simulink model "zcu216_tut_spec_cx"  (R2025a)
(part 2 of 76)

      mask TypeOptions t228_ref_clk: 923.077 | 857.143 | 800 | 750 | 705.882 | 666.667 | 631.579 | 600 | 571.429 | 545.455 | 521.739 | 500 | 480 | 461.538 | 444.444 | 428.571 | 413.793 | 400 | 387.097 | 375 | 363.636 | 352.941 | 342.857 | 333.333 | 324.324 | 315.789 | 307.692 | 300 | 292.683 | 285.714 | 279.07 | 272.727 | 266.667 | 260.87 | 255.319 | 250 | 244.898 | 240 | 235.294 | 230.769 | 226.415 | 222.222 | 218.182 | 214.286 | 210.526 | 206.897 | 203.39 | 200 | 196.721 | 193.548 | 190.476 | 187.5 | 184.615 | 181.818 | 179.104 | 176.471 | 173.913 | 171.429 | 169.014 | 166.667 | 164.384 | 162.162 | 160 | 157.895 | 155.844 | 153.846 | 151.899 | 150 | 148.148 | 146.341 | 144.578 | 142.857 | 141.176 | 139.535 | 137.931 | 136.364 | 134.831 | 133.333 | 131.868 | 130.435 | 129.032 | 127.66 | 126.316 | 125 | 123.711 | 122.449 | 121.212 | 120 | 118.812 | 117.647 | 116.505 | 115.385 | 114.286 | 113.208 | 112.15 | 111.111 | 110.092 | 109.091 | 108.108 | 107.143 | 106.195 | 105.263 | 104.348 | 103.448 | 102.564
      mask Callback t228_QT_dac0_enable: enable_dac_opt(gcb,228,0,'QT');
      mask TypeOptions t228_QT_dac0_analog_output: Real | I/Q
      mask Callback t228_QT_dac0_analog_output:
      | validate_analog_data(gcb,228,0,'QT');
      | update_axis_clk(gcb,228);
      mask TypeOptions t228_QT_dac0_inter_mode: 1x | 2x | 3x | 4x | 5x | 6x | 8x | 10x | 12x | 16x | 20x | 24x | 40x
      mask Callback t228_QT_dac0_inter_mode:
      | % if I/Q output mode, need to copy interp factor before updating axis clk
      | % note only the even slice for the tile makes this check
      | if chk_param(gcb, 't228_QT_dac0_analog_output', 'I/Q')
      |   inter_mode = get_param(gcb, 't228_QT_dac0_inter_mode');
      |   set_param(gcb, 't228_QT_dac1_inter_mode', inter_mode);
      | end
      | 
      | update_axis_clk(gcb,228);
      mask TypeOptions t228_QT_dac0_sample_per_cycle: 4 | 5 | 6 | 7 | 8 | 9 | 10 | 11 | 12 | 13 | 14 | 15 | 16
      mask Callback t228_QT_dac0_sample_per_cycle:
      | % if I/Q output mode, need to copy samples per clk before updating axis clk
      | if chk_param(gcb, 't228_QT_dac0_analog_output', 'I/Q')
      |   spc = get_param(gcb, 't228_QT_dac0_sample_per_cycle');
      |   set_param(gcb, 't228_QT_dac1_sample_per_cycle', spc);
      | end
      | 
      | update_axis_clk_label(gcb,228);
      mask TypeOptions t228_QT_dac0_datapath_mode: DUC 0 to Fs/2
      mask TypeOptions t228_QT_dac0_mixer_type: Coarse | Fine
      mask Callback t228_QT_dac0_mixer_type: mixertype_callback(gcb,228,0,'QT');
      mask TypeOptions t228_QT_dac0_mixer_mode: Real -> Real | I/Q -> Real
      mask Callback t228_QT_dac0_mixer_mode: mixer_callback(gcb,228,0,'QT');
      mask TypeOptions t228_QT_dac0_coarse_freq: 0
      mask TypeOptions t228_QT_dac0_nyquist_zone: Zone 1 | Zone 2
      mask TypeOptions t228_QT_dac0_decode_mode: SNR Optimized | Linearity Optimized
      mask Callback t228_QT_dac1_enable: enable_dac_opt(gcb,228,1,'QT');
      mask TypeOptions t228_QT_dac1_analog_output: Real | I/Q
      mask Callback t228_QT_dac1_analog_output:
      | validate_analog_data(gcb,228,1,'QT');
      | update_axis_clk(gcb,228);
      mask TypeOptions t228_QT_dac1_inter_mode: 1x | 2x | 3x | 4x | 5x | 6x | 8x | 10x | 12x | 16x | 20x | 24x | 40x
      mask Callback t228_QT_dac1_inter_mode: update_axis_clk(gcb,228);
      mask TypeOptions t228_QT_dac1_sample_per_cycle: 4 | 5 | 6 | 7 | 8 | 9 | 10 | 11 | 12 | 13 | 14 | 15 | 16
      mask Callback t228_QT_dac1_sample_per_cycle: update_axis_clk_label(gcb,228);
      mask TypeOptions t228_QT_dac1_datapath_mode: DUC 0 to Fs/2
      mask TypeOptions t228_QT_dac1_mixer_type: Coarse | Fine
      mask Callback t228_QT_dac1_mixer_type: mixertype_callback(gcb,228,1,'QT');
      mask TypeOptions t228_QT_dac1_mixer_mode: Real -> Real | I/Q -> Real
      mask Callback t228_QT_dac1_mixer_mode: mixer_callback(gcb,228,1,'QT')
      mask TypeOptions t228_QT_dac1_coarse_freq: 0
      mask TypeOptions t228_QT_dac1_nyquist_zone: Zone 1 | Zone 2
      mask TypeOptions t228_QT_dac1_decode_mode: SNR Optimized | Linearity Optimized
      mask Callback t228_QT_dac2_enable: enable_dac_opt(gcb,228,2,'QT');
      mask TypeOptions t228_QT_dac2_analog_output: Real | I/Q
      mask Callback t228_QT_dac2_analog_output:
      | validate_analog_data(gcb,228,2,'QT');
      | update_axis_clk(gcb,228);
      mask TypeOptions t228_QT_dac2_inter_mode: 1x | 2x | 3x | 4x | 5x | 6x | 8x | 10x | 12x | 16x | 20x | 24x | 40x
      mask Callback t228_QT_dac2_inter_mode:
      | % if I/Q output mode, need to copy interp factor before updating axis clk
      | % note only the even slice for the tile makes this check
      | if chk_param(gcb, 't228_QT_dac2_analog_output', 'I/Q')
      |   inter_mode = get_param(gcb, 't228_QT_dac2_inter_mode');
      |   set_param(gcb, 't228_QT_dac3_inter_mode', inter_mode);
      | end
      | update_axis_clk(gcb,228);
      mask TypeOptions t228_QT_dac2_sample_per_cycle: 4 | 5 | 6 | 7 | 8 | 9 | 10 | 11 | 12 | 13 | 14 | 15 | 16
      mask Callback t228_QT_dac2_sample_per_cycle:
      | % if I/Q output mode, need to copy samples per clk before updating axis clk
      | % note only the even slice for the tile makes this check
      | if chk_param(gcb, 't228_QT_dac2_analog_output', 'I/Q')
      |   spc = get_param(gcb, 't228_QT_dac2_sample_per_cycle');
      |   set_param(gcb, 't228_QT_dac3_sample_per_cycle', spc);
      | end
      | update_axis_clk_label(gcb,228);
      mask TypeOptions t228_QT_dac2_datapath_mode: DUC 0 to Fs/2
      mask TypeOptions t228_QT_dac2_mixer_type: Coarse | Fine
      mask Callback t228_QT_dac2_mixer_type: mixertype_callback(gcb,228,2,'QT');
      mask TypeOptions t228_QT_dac2_mixer_mode: Real -> Real | I/Q -> Real
      mask Callback t228_QT_dac2_mixer_mode: mixer_callback(gcb,228,2,'QT')
      mask TypeOptions t228_QT_dac2_coarse_freq: 0
      mask TypeOptions t228_QT_dac2_nyquist_zone: Zone 1 | Zone 2
      mask TypeOptions t228_QT_dac2_decode_mode: SNR Optimized | Linearity Optimized
      mask Callback t228_QT_dac3_enable: enable_dac_opt(gcb,228,3,'QT');
      mask TypeOptions t228_QT_dac3_analog_output: Real | I/Q
      mask Callback t228_QT_dac3_analog_output:
      | validate_analog_data(gcb,228,3,'QT');
      | update_axis_clk(gcb,228);
      mask TypeOptions t228_QT_dac3_inter_mode: 1x | 2x | 3x | 4x | 5x | 6x | 8x | 10x | 12x | 16x | 20x | 24x | 40x
      mask Callback t228_QT_dac3_inter_mode: update_axis_clk(gcb,228);
      mask TypeOptions t228_QT_dac3_sample_per_cycle: 4 | 5 | 6 | 7 | 8 | 9 | 10 | 11 | 12 | 13 | 14 | 15 | 16
      mask Callback t228_QT_dac3_sample_per_cycle: update_axis_clk_label(gcb,228);
      mask TypeOptions t228_QT_dac3_datapath_mode: DUC 0 to Fs/2
      mask TypeOptions t228_QT_dac3_mixer_type: Coarse | Fine
      mask Callback t228_QT_dac3_mixer_type: mixertype_callback(gcb,228,3,'QT');
      mask TypeOptions t228_QT_dac3_mixer_mode: Real -> Real | I/Q -> Real
      mask Callback t228_QT_dac3_mixer_mode: mixer_callback(gcb,228,3,'QT')
      mask TypeOptions t228_QT_dac3_coarse_freq: 0
      mask TypeOptions t228_QT_dac3_nyquist_zone: Zone 1 | Zone 2
      mask TypeOptions t228_QT_dac3_decode_mode: SNR Optimized | Linearity Optimized
      mask Callback t228_DT_dac0_enable: enable_dac_opt(gcb,228,0,'DT');
      mask TypeOptions t228_DT_dac0_analog_output: Real | I/Q
      mask Callback t228_DT_dac0_analog_output:
      | validate_analog_data(gcb,228,0,'DT');
      | update_axis_clk(gcb,228);
      mask TypeOptions t228_DT_dac0_inter_mode: 1x | 2x | 3x | 4x | 5x | 6x | 8x | 10x | 12x | 16x | 20x | 24x | 40x
      mask Callback t228_DT_dac0_inter_mode:
      | % if I/Q output mode, need to copy interp factor before updating axis clk
      | % note only the even slice for the tile makes this check
      | if chk_param(gcb, 't228_DT_dac0_analog_output', 'I/Q')
      |   inter_mode = get_param(gcb, 't228_DT_dac0_inter_mode');
      |   set_param(gcb, 't228_DT_dac1_inter_mode', inter_mode);
      | end
      | 
      | update_axis_clk(gcb,228);
      mask TypeOptions t228_DT_dac0_sample_per_cycle: 4 | 5 | 6 | 7 | 8 | 9 | 10 | 11 | 12 | 13 | 14 | 15 | 16
      mask Callback t228_DT_dac0_sample_per_cycle:
      | % if I/Q output mode, need to copy samples per clk before updating axis clk
      | if chk_param(gcb, 't228_DT_dac0_analog_output', 'I/Q')
      |   spc = get_param(gcb, 't228_DT_dac0_sample_per_cycle');
      |   set_param(gcb, 't228_DT_dac1_sample_per_cycle', spc);
      | end
      | update_axis_clk_label(gcb,228);
      mask TypeOptions t228_DT_dac0_datapath_mode: DUC 0 to Fs/2
      mask TypeOptions t228_DT_dac0_mixer_type: Coarse | Fine
      mask Callback t228_DT_dac0_mixer_type: mixertype_callback(gcb,228,0,'DT');
      mask TypeOptions t228_DT_dac0_mixer_mode: Real -> Real | I/Q -> Real
      mask Callback t228_DT_dac0_mixer_mode: mixer_callback(gcb,228,0,'DT');
      mask TypeOptions t228_DT_dac0_coarse_freq: 0
      mask TypeOptions t228_DT_dac0_nyquist_zone: Zone 1 | Zone 2
      mask TypeOptions t228_DT_dac0_decode_mode: SNR Optimized | Linearity Optimized
      mask Callback t228_DT_dac1_enable: enable_dac_opt(gcb,228,1,'DT');
      mask TypeOptions t228_DT_dac1_analog_output: Real
      mask Callback t228_DT_dac1_analog_output:
      | validate_analog_data(gcb,228,1,'DT');
      | update_axis_clk(gcb,228);
      mask TypeOptions t228_DT_dac1_inter_mode: 1x | 2x | 3x | 4x | 5x | 6x | 8x | 10x | 12x | 16x | 20x | 24x | 40x
      mask Callback t228_DT_dac1_inter_mode: update_axis_clk(gcb,228);
      mask TypeOptions t228_DT_dac1_sample_per_cycle: 4 | 5 | 6 | 7 | 8 | 9 | 10 | 11 | 12 | 13 | 14 | 15 | 16
      mask Callback t228_DT_dac1_sample_per_cycle:
      | %update_axis_clk(gcb);
      | update_axis_clk_label(gcb,228);
      mask TypeOptions t228_DT_dac1_datapath_mode: DUC 0 to Fs/2
      mask TypeOptions t228_DT_dac1_mixer_type: Coarse | Fine
      mask Callback t228_DT_dac1_mixer_type: mixertype_callback(gcb,228,1,'DT');
      mask TypeOptions t228_DT_dac1_mixer_mode: Real -> Real | I/Q -> Real
      mask Callback t228_DT_dac1_mixer_mode: mixer_callback(gcb,228,1,'DT');
      mask TypeOptions t228_DT_dac1_coarse_freq: 0
      mask TypeOptions t228_DT_dac1_nyquist_zone: Zone 1 | Zone 2
      mask TypeOptions t228_DT_dac1_decode_mode: SNR Optimized | Linearity Optimized
      mask Callback t229_sample_rate: update_rfdc_clocking(gcb,229);
      mask TypeOptions t229_clk_out: 125 | 62.5 | 31.25 | 15.625
      mask Callback t229_enable_pll:
      | %update_rfdc_clocking(gcb);
      | update_pll(gcb,229);
      mask TypeOptions t229_ref_clk: 923.077 | 857.143 | 800 | 750 | 705.882 | 666.667 | 631.579 | 600 | 571.429 | 545.455 | 521.739 | 500 | 480 | 461.538 | 444.444 | 428.571 | 413.793 | 400 | 387.097 | 375 | 363.636 | 352.941 | 342.857 | 333.333 | 324.324 | 315.789 | 307.692 | 300 | 292.683 | 285.714 | 279.07 | 272.727 | 266.667 | 260.87 | 255.319 | 250 | 244.898 | 240 | 235.294 | 230.769 | 226.415 | 222.222 | 218.182 | 214.286 | 210.526 | 206.897 | 203.39 | 200 | 196.721 | 193.548 | 190.476 | 187.5 | 184.615 | 181.818 | 179.104 | 176.471 | 173.913 | 171.429 | 169.014 | 166.667 | 164.384 | 162.162 | 160 | 157.895 | 155.844 | 153.846 | 151.899 | 150 | 148.148 | 146.341 | 144.578 | 142.857 | 141.176 | 139.535 | 137.931 | 136.364 | 134.831 | 133.333 | 131.868 | 130.435 | 129.032 | 127.66 | 126.316 | 125 | 123.711 | 122.449 | 121.212 | 120 | 118.812 | 117.647 | 116.505 | 115.385 | 114.286 | 113.208 | 112.15 | 111.111 | 110.092 | 109.091 | 108.108 | 107.143 | 106.195 | 105.263 | 104.348 | 103.448 | 102.564
      mask Callback t229_QT_dac0_enable: enable_dac_opt(gcb,229,0,'QT');
      mask TypeOptions t229_QT_dac0_analog_output: Real | I/Q
      mask Callback t229_QT_dac0_analog_output:
      | validate_analog_data(gcb,229,0,'QT');
      | update_axis_clk(gcb,229);
      mask TypeOptions t229_QT_dac0_inter_mode: 1x | 2x | 3x | 4x | 5x | 6x | 8x | 10x | 12x | 16x | 20x | 24x | 40x
      mask Callback t229_QT_dac0_inter_mode:
      | % if I/Q output mode, need to copy interp factor before updating axis clk
      | % note only the even slice for the tile makes this check
      | if chk_param(gcb, 't229_QT_dac0_analog_output', 'I/Q')
      |   inter_mode = get_param(gcb, 't229_QT_dac0_inter_mode');
      |   set_param(gcb, 't229_QT_dac1_inter_mode', inter_mode);
      | end
      | update_axis_clk(gcb,229);
      mask TypeOptions t229_QT_dac0_sample_per_cycle: 4 | 5 | 6 | 7 | 8 | 9 | 10 | 11 | 12 | 13 | 14 | 15 | 16
      mask Callback t229_QT_dac0_sample_per_cycle:
      | % if I/Q output mode, need to copy samples per clk before updating axis clk
      | % note only the even slice for the tile makes this check
      | if chk_param(gcb, 't229_QT_dac0_analog_output', 'I/Q')
      |   spc = get_param(gcb, 't229_QT_dac0_sample_per_cycle');
      |   set_param(gcb, 't229_QT_dac1_sample_per_cycle', spc);
      | end
      | update_axis_clk_label(gcb,229);
      mask TypeOptions t229_QT_dac0_datapath_mode: DUC 0 to Fs/2
      mask TypeOptions t229_QT_dac0_mixer_type: Coarse | Fine
      mask Callback t229_QT_dac0_mixer_type: mixertype_callback(gcb,229,0,'QT');
      mask TypeOptions t229_QT_dac0_mixer_mode: Real -> Real | I/Q -> Real
      mask Callback t229_QT_dac0_mixer_mode: mixer_callback(gcb,229,0,'QT');
      mask TypeOptions t229_QT_dac0_coarse_freq: 0
      mask TypeOptions t229_QT_dac0_nyquist_zone: Zone 1 | Zone 2
      mask TypeOptions t229_QT_dac0_decode_mode: SNR Optimized | Linearity Optimized
      mask Callback t229_QT_dac1_enable: enable_dac_opt(gcb,229,1,'QT');
      mask TypeOptions t229_QT_dac1_analog_output: Real
      mask Callback t229_QT_dac1_analog_output:
      | validate_analog_data(gcb,229,1,'QT');
      | update_axis_clk(gcb,229);
      mask TypeOptions t229_QT_dac1_inter_mode: 1x | 2x | 3x | 4x | 5x | 6x | 8x | 10x | 12x | 16x | 20x | 24x | 40x
      mask Callback t229_QT_dac1_inter_mode: update_axis_clk(gcb,229);
      mask TypeOptions t229_QT_dac1_sample_per_cycle: 4 | 5 | 6 | 7 | 8 | 9 | 10 | 11 | 12 | 13 | 14 | 15 | 16
      mask Callback t229_QT_dac1_sample_per_cycle: update_axis_clk_label(gcb,229);
      mask TypeOptions t229_QT_dac1_datapath_mode: DUC 0 to Fs/2
      mask TypeOptions t229_QT_dac1_mixer_type: Coarse | Fine
      mask Callback t229_QT_dac1_mixer_type: mixertype_callback(gcb,229,1,'QT');
      mask TypeOptions t229_QT_dac1_mixer_mode: Real -> Real | I/Q -> Real
      mask Callback t229_QT_dac1_mixer_mode: mixer_callback(gcb,229,1,'QT')
      mask TypeOptions t229_QT_dac1_coarse_freq: 0
      mask TypeOptions t229_QT_dac1_nyquist_zone: Zone 1 | Zone 2
      mask TypeOptions t229_QT_dac1_decode_mode: SNR Optimized | Linearity Optimized
      mask Callback t229_QT_dac2_enable: enable_dac_opt(gcb,229,2,'QT');
      mask TypeOptions t229_QT_dac2_analog_output: Real | I/Q
      mask Callback t229_QT_dac2_analog_output:
      | validate_analog_data(gcb,229,2,'QT');
      | update_axis_clk(gcb,229);
      mask TypeOptions t229_QT_dac2_inter_mode: 1x | 2x | 3x | 4x | 5x | 6x | 8x | 10x | 12x | 16x | 20x | 24x | 40x
      mask Callback t229_QT_dac2_inter_mode:
      | % if I/Q output mode, need to copy interp factor before updating axis clk
      | % note only the even slice for the tile makes this check
      | if chk_param(gcb, 't229_QT_dac2_analog_output', 'I/Q')
      |   inter_mode = get_param(gcb, 't229_QT_dac2_inter_mode');
      |   set_param(gcb, 't229_QT_dac3_inter_mode', inter_mode);
      | end
      | update_axis_clk(gcb,229);
      mask TypeOptions t229_QT_dac2_sample_per_cycle: 4 | 5 | 6 | 7 | 8 | 9 | 10 | 11 | 12 | 13 | 14 | 15 | 16
      mask Callback t229_QT_dac2_sample_per_cycle:
      | % if I/Q output mode, need to copy samples per clk before updating axis clk
      | % note only the even slice for the tile makes this check
      | if chk_param(gcb, 't229_QT_dac2_analog_output', 'I/Q')
      |   spc = get_param(gcb, 't229_QT_dac2_sample_per_cycle');
      |   set_param(gcb, 't229_QT_dac3_sample_per_cycle', spc);
      | end
      | update_axis_clk_label(gcb,229);
      mask TypeOptions t229_QT_dac2_datapath_mode: DUC 0 to Fs/2
      mask TypeOptions t229_QT_dac2_mixer_type: Coarse | Fine
      mask Callback t229_QT_dac2_mixer_type: mixertype_callback(gcb,229,2,'QT');
      mask TypeOptions t229_QT_dac2_mixer_mode: Real -> Real | I/Q -> Real
      mask Callback t229_QT_dac2_mixer_mode: mixer_callback(gcb,229,2,'QT')
      mask TypeOptions t229_QT_dac2_coarse_freq: 0
      mask TypeOptions t229_QT_dac2_nyquist_zone: Zone 1 | Zone 2
      mask TypeOptions t229_QT_dac2_decode_mode: SNR Optimized | Linearity Optimized
      mask Callback t229_QT_dac3_enable: enable_dac_opt(gcb,229,3,'QT');
      mask TypeOptions t229_QT_dac3_analog_output: Real | I/Q
      mask Callback t229_QT_dac3_analog_output:
      | validate_analog_data(gcb,229,3,'QT');
      | update_axis_clk(gcb,229);
      mask TypeOptions t229_QT_dac3_inter_mode: 1x | 2x | 3x | 4x | 5x | 6x | 8x | 10x | 12x | 16x | 20x | 24x | 40x
      mask Callback t229_QT_dac3_inter_mode: update_axis_clk(gcb,229);
      mask TypeOptions t229_QT_dac3_sample_per_cycle: 4 | 5 | 6 | 7 | 8 | 9 | 10 | 11 | 12 | 13 | 14 | 15 | 16
      mask Callback t229_QT_dac3_sample_per_cycle: update_axis_clk_label(gcb,229);
      mask TypeOptions t229_QT_dac3_datapath_mode: DUC 0 to Fs/2
      mask TypeOptions t229_QT_dac3_mixer_type: Coarse | Fine
      mask Callback t229_QT_dac3_mixer_type: mixertype_callback(gcb,229,3,'QT');
      mask TypeOptions t229_QT_dac3_mixer_mode: Real -> Real | I/Q -> Real
      mask Callback t229_QT_dac3_mixer_mode: mixer_callback(gcb,229,3,'QT')
      mask TypeOptions t229_QT_dac3_coarse_freq: 0
      mask TypeOptions t229_QT_dac3_nyquist_zone: Zone 1 | Zone 2
      mask TypeOptions t229_QT_dac3_decode_mode: SNR Optimized | Linearity Optimized
      mask Callback t229_DT_dac0_enable: enable_dac_opt(gcb,229,0,'DT');
      mask TypeOptions t229_DT_dac0_analog_output: Real | I/Q
      mask Callback t229_DT_dac0_analog_output:
      | validate_analog_data(gcb,229,0,'DT');
      | update_axis_clk(gcb,229);
      mask TypeOptions t229_DT_dac0_inter_mode: 1x | 2x | 3x | 4x | 5x | 6x | 8x | 10x | 12x | 16x | 20x | 24x | 40x
      mask Callback t229_DT_dac0_inter_mode:
      | % if I/Q output mode, need to copy interp factor before updating axis clk
      | % note only the even slice for the tile makes this check
      | if chk_param(gcb, 't229_DT_dac0_analog_output', 'I/Q')
      |   inter_mode = get_param(gcb, 't229_DT_dac0_inter_mode');
      |   set_param(gcb, 't229_DT_dac1_inter_mode', inter_mode);
      | end
      | update_axis_clk(gcb,229);
      mask TypeOptions t229_DT_dac0_sample_per_cycle: 4 | 5 | 6 | 7 | 8 | 9 | 10 | 11 | 12 | 13 | 14 | 15 | 16
      mask Callback t229_DT_dac0_sample_per_cycle:
      | % if I/Q output mode, need to copy samples per clk before updating axis clk
      | % note only the even slice for the tile makes this check
      | if chk_param(gcb, 't229_DT_dac0_analog_output', 'I/Q')
      |   spc = get_param(gcb, 't229_DT_dac0_sample_per_cycle');
      |   set_param(gcb, 't229_DT_dac1_sample_per_cycle', spc);
      | end
      | update_axis_clk_label(gcb,229);
      mask TypeOptions t229_DT_dac0_datapath_mode: DUC 0 to Fs/2
      mask TypeOptions t229_DT_dac0_mixer_type: Coarse | Fine
      mask Callback t229_DT_dac0_mixer_type: mixertype_callback(gcb,229,0,'DT');
      mask TypeOptions t229_DT_dac0_mixer_mode: Real -> Real | I/Q -> Real
      mask Callback t229_DT_dac0_mixer_mode: mixer_callback(gcb,229,0,'DT');
      mask TypeOptions t229_DT_dac0_coarse_freq: 0
      mask TypeOptions t229_DT_dac0_nyquist_zone: Zone 1 | Zone 2
      mask TypeOptions t229_DT_dac0_decode_mode: SNR Optimized | Linearity Optimized
      mask Callback t229_DT_dac1_enable: enable_dac_opt(gcb,229,1,'DT');
      mask TypeOptions t229_DT_dac1_analog_output: Real
      mask Callback t229_DT_dac1_analog_output:
      | validate_analog_data(gcb,229,1,'DT');
      | update_axis_clk(gcb,229);
      mask TypeOptions t229_DT_dac1_inter_mode: 1x | 2x | 3x | 4x | 5x | 6x | 8x | 10x | 12x | 16x | 20x | 24x | 40x
      mask Callback t229_DT_dac1_inter_mode: update_axis_clk(gcb,229);
      mask TypeOptions t229_DT_dac1_sample_per_cycle: 4 | 5 | 6 | 7 | 8 | 9 | 10 | 11 | 12 | 13 | 14 | 15 | 16
      mask Callback t229_DT_dac1_sample_per_cycle:
      | %update_axis_clk(gcb);
      | update_axis_clk_label(gcb,229);
      mask TypeOptions t229_DT_dac1_datapath_mode: DUC 0 to Fs/2
      mask TypeOptions t229_DT_dac1_mixer_type: Coarse | Fine
      mask Callback t229_DT_dac1_mixer_type: mixertype_callback(gcb,229,1,'DT');
      mask TypeOptions t229_DT_dac1_mixer_mode: Real -> Real | I/Q -> Real
      mask Callback t229_DT_dac1_mixer_mode: mixer_callback(gcb,229,1,'DT');
      mask TypeOptions t229_DT_dac1_coarse_freq: 0
      mask TypeOptions t229_DT_dac1_nyquist_zone: Zone 1 | Zone 2
      mask TypeOptions t229_DT_dac1_decode_mode: SNR Optimized | Linearity Optimized
      mask Callback t230_sample_rate: update_rfdc_clocking(gcb,230);
      mask TypeOptions t230_clk_out: 125 | 62.5 | 31.25 | 15.625
      mask Callback t230_enable_pll:
      | %update_rfdc_clocking(gcb);
      | update_pll(gcb,230);
      mask TypeOptions t230_ref_clk: 923.077 | 857.143 | 800 | 750 | 705.882 | 666.667 | 631.579 | 600 | 571.429 | 545.455 | 521.739 | 500 | 480 | 461.538 | 444.444 | 428.571 | 413.793 | 400 | 387.097 | 375 | 363.636 | 352.941 | 342.857 | 333.333 | 324.324 | 315.789 | 307.692 | 300 | 292.683 | 285.714 | 279.07 | 272.727 | 266.667 | 260.87 | 255.319 | 250 | 244.898 | 240 | 235.294 | 230.769 | 226.415 | 222.222 | 218.182 | 214.286 | 210.526 | 206.897 | 203.39 | 200 | 196.721 | 193.548 | 190.476 | 187.5 | 184.615 | 181.818 | 179.104 | 176.471 | 173.913 | 171.429 | 169.014 | 166.667 | 164.384 | 162.162 | 160 | 157.895 | 155.844 | 153.846 | 151.899 | 150 | 148.148 | 146.341 | 144.578 | 142.857 | 141.176 | 139.535 | 137.931 | 136.364 | 134.831 | 133.333 | 131.868 | 130.435 | 129.032 | 127.66 | 126.316 | 125 | 123.711 | 122.449 | 121.212 | 120 | 118.812 | 117.647 | 116.505 | 115.385 | 114.286 | 113.208 | 112.15 | 111.111 | 110.092 | 109.091 | 108.108 | 107.143 | 106.195 | 105.263 | 104.348 | 103.448 | 102.564
      mask Callback t230_QT_dac0_enable: enable_dac_opt(gcb,230,0,'QT');
      mask TypeOptions t230_QT_dac0_analog_output: Real | I/Q
      mask Callback t230_QT_dac0_analog_output:
      | validate_analog_data(gcb,230,0,'QT');
      | update_axis_clk(gcb,230);
      mask TypeOptions t230_QT_dac0_inter_mode: 1x | 2x | 3x | 4x | 5x | 6x | 8x | 10x | 12x | 16x | 20x | 24x | 40x
      mask Callback t230_QT_dac0_inter_mode:
      | % if I/Q output mode, need to copy interp factor before updating axis clk
      | % note only the even slice for the tile makes this check
      | if chk_param(gcb, 't230_QT_dac0_analog_output', 'I/Q')
      |   inter_mode = get_param(gcb, 't230_QT_dac0_inter_mode');
      |   set_param(gcb, 't230_QT_dac1_inter_mode', inter_mode);
      | end
      | update_axis_clk(gcb,230);
      mask TypeOptions t230_QT_dac0_sample_per_cycle: 4 | 5 | 6 | 7 | 8 | 9 | 10 | 11 | 12 | 13 | 14 | 15 | 16
      mask Callback t230_QT_dac0_sample_per_cycle:
      | % if I/Q output mode, need to copy samples per clk before updating axis clk
      | % note only the even slice for the tile makes this check
      | if chk_param(gcb, 't230_QT_dac0_analog_output', 'I/Q')
      |   spc = get_param(gcb, 't230_QT_dac0_sample_per_cycle');
      |   set_param(gcb, 't230_QT_dac1_sample_per_cycle', spc);
      | end
      | 
      | update_axis_clk_label(gcb,230);
      mask TypeOptions t230_QT_dac0_datapath_mode: DUC 0 to Fs/2
      mask TypeOptions t230_QT_dac0_mixer_type: Coarse | Fine
      mask Callback t230_QT_dac0_mixer_type: mixertype_callback(gcb,230,0,'QT');
      mask TypeOptions t230_QT_dac0_mixer_mode: Real -> Real | I/Q -> Real
      mask Callback t230_QT_dac0_mixer_mode: mixer_callback(gcb,230,0,'QT');
      mask TypeOptions t230_QT_dac0_coarse_freq: 0
      mask TypeOptions t230_QT_dac0_nyquist_zone: Zone 1 | Zone 2
      mask TypeOptions t230_QT_dac0_decode_mode: SNR Optimized | Linearity Optimized
      mask Callback t230_QT_dac1_enable: enable_dac_opt(gcb,230,1,'QT');
      mask TypeOptions t230_QT_dac1_analog_output: Real | I/Q
      mask Callback t230_QT_dac1_analog_output:
      | validate_analog_data(gcb,230,1,'QT');
      | update_axis_clk(gcb,230);
      mask TypeOptions t230_QT_dac1_inter_mode: 1x | 2x | 3x | 4x | 5x | 6x | 8x | 10x | 12x | 16x | 20x | 24x | 40x
      mask Callback t230_QT_dac1_inter_mode: update_axis_clk(gcb,230);
      mask TypeOptions t230_QT_dac1_sample_per_cycle: 4 | 5 | 6 | 7 | 8 | 9 | 10 | 11 | 12 | 13 | 14 | 15 | 16
      mask Callback t230_QT_dac1_sample_per_cycle: update_axis_clk_label(gcb,230);
      mask TypeOptions t230_QT_dac1_datapath_mode: DUC 0 to Fs/2
      mask TypeOptions t230_QT_dac1_mixer_type: Coarse | Fine
      mask Callback t230_QT_dac1_mixer_type: mixertype_callback(gcb,230,1,'QT');
      mask TypeOptions t230_QT_dac1_mixer_mode: Real -> Real | I/Q -> Real
      mask Callback t230_QT_dac1_mixer_mode: mixer_callback(gcb,230,1,'QT')
      mask TypeOptions t230_QT_dac1_coarse_freq: 0
      mask TypeOptions t230_QT_dac1_nyquist_zone: Zone 1 | Zone 2
      mask TypeOptions t230_QT_dac1_decode_mode: SNR Optimized | Linearity Optimized
      mask Callback t230_QT_dac2_enable: enable_dac_opt(gcb,230,2,'QT');
      mask TypeOptions t230_QT_dac2_analog_output: Real | I/Q
      mask Callback t230_QT_dac2_analog_output:
      | validate_analog_data(gcb,230,2,'QT');
      | update_axis_clk(gcb,230);
      mask TypeOptions t230_QT_dac2_inter_mode: 1x | 2x | 3x | 4x | 5x | 6x | 8x | 10x | 12x | 16x | 20x | 24x | 40x
      mask Callback t230_QT_dac2_inter_mode:
      | % if I/Q output mode, need to copy interp factor before updating axis clk
      | % note only the even slice for the tile makes this check
      | if chk_param(gcb, 't230_QT_dac2_analog_output', 'I/Q')
      |   inter_mode = get_param(gcb, 't230_QT_dac2_inter_mode');
      |   set_param(gcb, 't230_QT_dac3_inter_mode', inter_mode);
      | end
      | 
      | update_axis_clk(gcb,230);
      mask TypeOptions t230_QT_dac2_sample_per_cycle: 4 | 5 | 6 | 7 | 8 | 9 | 10 | 11 | 12 | 13 | 14 | 15 | 16
      mask Callback t230_QT_dac2_sample_per_cycle:
      | % if I/Q output mode, need to copy samples per clk before updating axis clk
      | % note only the even slice for the tile makes this check
      | if chk_param(gcb, 't230_QT_dac2_analog_output', 'I/Q')
      |   spc = get_param(gcb, 't230_QT_dac2_sample_per_cycle');
      |   set_param(gcb, 't230_QT_dac3_sample_per_cycle', spc);
      | end
      | 
      | update_axis_clk_label(gcb,230)
      mask TypeOptions t230_QT_dac2_datapath_mode: DUC 0 to Fs/2
      mask TypeOptions t230_QT_dac2_mixer_type: Coarse | Fine
      mask Callback t230_QT_dac2_mixer_type: mixertype_callback(gcb,230,2,'QT');
      mask TypeOptions t230_QT_dac2_mixer_mode: Real -> Real | I/Q -> Real
      mask Callback t230_QT_dac2_mixer_mode: mixer_callback(gcb,230,2,'QT')
      mask TypeOptions t230_QT_dac2_coarse_freq: 0
      mask TypeOptions t230_QT_dac2_nyquist_zone: Zone 1 | Zone 2
      mask TypeOptions t230_QT_dac2_decode_mode: SNR Optimized | Linearity Optimized
      mask Callback t230_QT_dac3_enable: enable_dac_opt(gcb,230,3,'QT');
      mask TypeOptions t230_QT_dac3_analog_output: Real | I/Q
      mask Callback t230_QT_dac3_analog_output:
      | validate_analog_data(gcb,230,3,'QT');
      | update_axis_clk(gcb,230);
      mask TypeOptions t230_QT_dac3_inter_mode: 1x | 2x | 3x | 4x | 5x | 6x | 8x | 10x | 12x | 16x | 20x | 24x | 40x
      mask Callback t230_QT_dac3_inter_mode: update_axis_clk(gcb,230);
      mask TypeOptions t230_QT_dac3_sample_per_cycle: 4 | 5 | 6 | 7 | 8 | 9 | 10 | 11 | 12 | 13 | 14 | 15 | 16
      mask Callback t230_QT_dac3_sample_per_cycle: update_axis_clk_label(gcb,230);
      mask TypeOptions t230_QT_dac3_datapath_mode: DUC 0 to Fs/2
      mask TypeOptions t230_QT_dac3_mixer_type: Coarse | Fine
      mask Callback t230_QT_dac3_mixer_type: mixertype_callback(gcb,230,3,'QT');
      mask TypeOptions t230_QT_dac3_mixer_mode: Real -> Real | I/Q -> Real
      mask Callback t230_QT_dac3_mixer_mode: mixer_callback(gcb,230,3,'QT')
      mask TypeOptions t230_QT_dac3_coarse_freq: 0
      mask TypeOptions t230_QT_dac3_nyquist_zone: Zone 1 | Zone 2
      mask TypeOptions t230_QT_dac3_decode_mode: SNR Optimized | Linearity Optimized
      mask Callback t230_DT_dac0_enable: enable_dac_opt(gcb,230,0,'DT');
      mask TypeOptions t230_DT_dac0_analog_output: Real | I/Q
      mask Callback t230_DT_dac0_analog_output:
      | validate_analog_data(gcb,230,0,'DT');
      | update_axis_clk(gcb,230);
      mask TypeOptions t230_DT_dac0_inter_mode: 1x | 2x | 3x | 4x | 5x | 6x | 8x | 10x | 12x | 16x | 20x | 24x | 40x
      mask Callback t230_DT_dac0_inter_mode:
      | % if I/Q output mode, need to copy interp factor before updating axis clk
      | % note only the even slice for the tile makes this check
      | if chk_param(gcb, 't230_DT_dac0_analog_output', 'I/Q')
      |   inter_mode = get_param(gcb, 't230_DT_dac0_inter_mode');
      |   set_param(gcb, 't230_DT_dac1_inter_mode', inter_mode);
      | end
      | 
      | update_axis_clk(gcb,230);
      mask TypeOptions t230_DT_dac0_sample_per_cycle: 4 | 5 | 6 | 7 | 8 | 9 | 10 | 11 | 12 | 13 | 14 | 15 | 16
      mask Callback t230_DT_dac0_sample_per_cycle:
      | % if I/Q output mode, need to copy samples per clk before updating axis clk
      | % note only the even slice for the tile makes this check
      | if chk_param(gcb, 't230_DT_dac0_analog_output', 'I/Q')
      |   spc = get_param(gcb, 't230_DT_dac0_sample_per_cycle');
      |   set_param(gcb, 't230_DT_dac1_sample_per_cycle', spc);
      | end
      | update_axis_clk_label(gcb,230);
      mask TypeOptions t230_DT_dac0_datapath_mode: DUC 0 to Fs/2
      mask TypeOptions t230_DT_dac0_mixer_type: Coarse | Fine
      mask Callback t230_DT_dac0_mixer_type: mixertype_callback(gcb,230,0,'DT');
      mask TypeOptions t230_DT_dac0_mixer_mode: Real -> Real | I/Q -> Real
      mask Callback t230_DT_dac0_mixer_mode: mixer_callback(gcb,230,0,'DT');
      mask TypeOptions t230_DT_dac0_coarse_freq: 0
      mask TypeOptions t230_DT_dac0_nyquist_zone: Zone 1 | Zone 2
      mask TypeOptions t230_DT_dac0_decode_mode: SNR Optimized | Linearity Optimized
      mask Callback t230_DT_dac1_enable: enable_dac_opt(gcb,230,1,'DT');
      mask TypeOptions t230_DT_dac1_analog_output: Real
      mask Callback t230_DT_dac1_analog_output:
      | validate_analog_data(gcb,230,1,'DT');
      | update_axis_clk(gcb,229);
      mask TypeOptions t230_DT_dac1_inter_mode: 1x | 2x | 3x | 4x | 5x | 6x | 8x | 10x | 12x | 16x | 20x | 24x | 40x
      mask Callback t230_DT_dac1_inter_mode: update_axis_clk(gcb,230);
      mask TypeOptions t230_DT_dac1_sample_per_cycle: 4 | 5 | 6 | 7 | 8 | 9 | 10 | 11 | 12 | 13 | 14 | 15 | 16
      mask Callback t230_DT_dac1_sample_per_cycle:
      | %update_axis_clk(gcb);
      | update_axis_clk_label(gcb,230);
      mask TypeOptions t230_DT_dac1_datapath_mode: DUC 0 to Fs/2
      mask TypeOptions t230_DT_dac1_mixer_type: Coarse | Fine
      mask Callback t230_DT_dac1_mixer_type: mixertype_callback(gcb,230,1,'DT');
      mask TypeOptions t230_DT_dac1_mixer_mode: Real -> Real | I/Q -> Real
      mask Callback t230_DT_dac1_mixer_mode: mixer_callback(gcb,230,1,'DT');
      mask TypeOptions t230_DT_dac1_coarse_freq: 0
      mask TypeOptions t230_DT_dac1_nyquist_zone: Zone 1 | Zone 2
      mask TypeOptions t230_DT_dac1_decode_mode: SNR Optimized | Linearity Optimized
      mask Callback t231_sample_rate: update_rfdc_clocking(gcb,231);
      mask TypeOptions t231_clk_out: 125 | 62.5 | 31.25 | 15.625
      mask Callback t231_enable_pll:
      | %update_rfdc_clocking(gcb);
      | update_pll(gcb,231);
      mask TypeOptions t231_ref_clk: 923.077 | 857.143 | 800 | 750 | 705.882 | 666.667 | 631.579 | 600 | 571.429 | 545.455 | 521.739 | 500 | 480 | 461.538 | 444.444 | 428.571 | 413.793 | 400 | 387.097 | 375 | 363.636 | 352.941 | 342.857 | 333.333 | 324.324 | 315.789 | 307.692 | 300 | 292.683 | 285.714 | 279.07 | 272.727 | 266.667 | 260.87 | 255.319 | 250 | 244.898 | 240 | 235.294 | 230.769 | 226.415 | 222.222 | 218.182 | 214.286 | 210.526 | 206.897 | 203.39 | 200 | 196.721 | 193.548 | 190.476 | 187.5 | 184.615 | 181.818 | 179.104 | 176.471 | 173.913 | 171.429 | 169.014 | 166.667 | 164.384 | 162.162 | 160 | 157.895 | 155.844 | 153.846 | 151.899 | 150 | 148.148 | 146.341 | 144.578 | 142.857 | 141.176 | 139.535 | 137.931 | 136.364 | 134.831 | 133.333 | 131.868 | 130.435 | 129.032 | 127.66 | 126.316 | 125 | 123.711 | 122.449 | 121.212 | 120 | 118.812 | 117.647 | 116.505 | 115.385 | 114.286 | 113.208 | 112.15 | 111.111 | 110.092 | 109.091 | 108.108 | 107.143 | 106.195 | 105.263 | 104.348 | 103.448 | 102.564
      mask Callback t231_QT_dac0_enable: enable_dac_opt(gcb,231,0,'QT');
      mask TypeOptions t231_QT_dac0_analog_output: Real | I/Q
      mask Callback t231_QT_dac0_analog_output:
      | validate_analog_data(gcb,231,0,'QT');
      | update_axis_clk(gcb,231);
      mask TypeOptions t231_QT_dac0_inter_mode: 1x | 2x | 3x | 4x | 5x | 6x | 8x | 10x | 12x | 16x | 20x | 24x | 40x
      mask Callback t231_QT_dac0_inter_mode:
      | % if I/Q output mode, need to copy interp factor before updating axis clk
      | % note only the even slice for the tile makes this check
      | if chk_param(gcb, 't231_QT_dac0_analog_output', 'I/Q')
      |   inter_mode = get_param(gcb, 't231_QT_dac0_inter_mode');
      |   set_param(gcb, 't231_QT_dac1_inter_mode', inter_mode);
      | end
      | update_axis_clk(gcb,231);
      mask TypeOptions t231_QT_dac0_sample_per_cycle: 4 | 5 | 6 | 7 | 8 | 9 | 10 | 11 | 12 | 13 | 14 | 15 | 16
      mask Callback t231_QT_dac0_sample_per_cycle:
      | % if I/Q output mode, need to copy samples per clk before updating axis clk
      | % note only the even slice for the tile makes this check
      | if chk_param(gcb, 't231_QT_dac0_analog_output', 'I/Q')
      |   spc = get_param(gcb, 't231_QT_dac0_sample_per_cycle');
      |   set_param(gcb, 't231_QT_dac1_sample_per_cycle', spc);
      | end
      | update_axis_clk_label(gcb,231);
      mask TypeOptions t231_QT_dac0_datapath_mode: DUC 0 to Fs/2
      mask TypeOptions t231_QT_dac0_mixer_type: Coarse | Fine
      mask Callback t231_QT_dac0_mixer_type: mixertype_callback(gcb,231,0,'QT');
      mask TypeOptions t231_QT_dac0_mixer_mode: Real -> Real | I/Q -> Real
      mask Callback t231_QT_dac0_mixer_mode: mixer_callback(gcb,231,0,'QT');
      mask TypeOptions t231_QT_dac0_coarse_freq: 0
      mask TypeOptions t231_QT_dac0_nyquist_zone: Zone 1 | Zone 2
      mask TypeOptions t231_QT_dac0_decode_mode: SNR Optimized | Linearity Optimized
      mask Callback t231_QT_dac1_enable: enable_dac_opt(gcb,231,1,'QT');
      mask TypeOptions t231_QT_dac1_analog_output: Real | I/Q
      mask Callback t231_QT_dac1_analog_output:
      | validate_analog_data(gcb,231,1,'QT');
      | update_axis_clk(gcb,231);
      mask TypeOptions t231_QT_dac1_inter_mode: 1x | 2x | 3x | 4x | 5x | 6x | 8x | 10x | 12x | 16x | 20x | 24x | 40x
      mask Callback t231_QT_dac1_inter_mode: update_axis_clk(gcb,231);
      mask TypeOptions t231_QT_dac1_sample_per_cycle: 4 | 5 | 6 | 7 | 8 | 9 | 10 | 11 | 12 | 13 | 14 | 15 | 16
      mask Callback t231_QT_dac1_sample_per_cycle: update_axis_clk_label(gcb,231);
      mask TypeOptions t231_QT_dac1_datapath_mode: DUC 0 to Fs/2
      mask TypeOptions t231_QT_dac1_mixer_type: Coarse | Fine
      mask Callback t231_QT_dac1_mixer_type: mixertype_callback(gcb,231,1,'QT');
      mask TypeOptions t231_QT_dac1_mixer_mode: Real -> Real | I/Q -> Real
      mask Callback t231_QT_dac1_mixer_mode: mixer_callback(gcb,231,1,'QT')
      mask TypeOptions t231_QT_dac1_coarse_freq: 0
      mask TypeOptions t231_QT_dac1_nyquist_zone: Zone 1 | Zone 2
      mask TypeOptions t231_QT_dac1_decode_mode: SNR Optimized | Linearity Optimized
      mask Callback t231_QT_dac2_enable: enable_dac_opt(gcb,231,2,'QT');
      mask TypeOptions t231_QT_dac2_analog_output: Real | I/Q
      mask Callback t231_QT_dac2_analog_output:
      | validate_analog_data(gcb,231,2,'QT');
      | update_axis_clk(gcb,231);
      mask TypeOptions t231_QT_dac2_inter_mode: 1x | 2x | 3x | 4x | 5x | 6x | 8x | 10x | 12x | 16x | 20x | 24x | 40x
      mask Callback t231_QT_dac2_inter_mode:
      | % if I/Q output mode, need to copy interp factor before updating axis clk
      | % note only the even slice for the tile makes this check
      | if chk_param(gcb, 't231_QT_dac2_analog_output', 'I/Q')
      |   inter_mode = get_param(gcb, 't231_QT_dac2_inter_mode');
      |   set_param(gcb, 't231_QT_dac3_inter_mode', inter_mode);
      | end
      | update_axis_clk(gcb,231);
      mask TypeOptions t231_QT_dac2_sample_per_cycle: 4 | 5 | 6 | 7 | 8 | 9 | 10 | 11 | 12 | 13 | 14 | 15 | 16
      mask Callback t231_QT_dac2_sample_per_cycle:
      | % if I/Q output mode, need to copy samples per clk before updating axis clk
      | % note only the even slice for the tile makes this check
      | if chk_param(gcb, 't231_QT_dac2_analog_output', 'I/Q')
      |   spc = get_param(gcb, 't231_QT_dac2_sample_per_cycle');
      |   set_param(gcb, 't231_QT_dac3_sample_per_cycle', spc);
      | end
      | update_axis_clk_label(gcb,231);
      mask TypeOptions t231_QT_dac2_datapath_mode: DUC 0 to Fs/2
      mask TypeOptions t231_QT_dac2_mixer_type: Coarse | Fine
      mask Callback t231_QT_dac2_mixer_type: mixertype_callback(gcb,231,2,'QT');
      mask TypeOptions t231_QT_dac2_mixer_mode: Real -> Real | I/Q -> Real
      mask Callback t231_QT_dac2_mixer_mode: mixer_callback(gcb,231,2,'QT')
      mask TypeOptions t231_QT_dac2_coarse_freq: 0
      mask TypeOptions t231_QT_dac2_nyquist_zone: Zone 1 | Zone 2
      mask TypeOptions t231_QT_dac2_decode_mode: SNR Optimized | Linearity Optimized
      mask Callback t231_QT_dac3_enable: enable_dac_opt(gcb,231,3,'QT');
      mask TypeOptions t231_QT_dac3_analog_output: Real | I/Q
      mask Callback t231_QT_dac3_analog_output:
      | validate_analog_data(gcb,231,3,'QT');
      | update_axis_clk(gcb,231);
      mask TypeOptions t231_QT_dac3_inter_mode: 1x | 2x | 3x | 4x | 5x | 6x | 8x | 10x | 12x | 16x | 20x | 24x | 40x
      mask Callback t231_QT_dac3_inter_mode: update_axis_clk(gcb,231);
      mask TypeOptions t231_QT_dac3_sample_per_cycle: 4 | 5 | 6 | 7 | 8 | 9 | 10 | 11 | 12 | 13 | 14 | 15 | 16
      mask Callback t231_QT_dac3_sample_per_cycle: update_axis_clk_label(gcb,231);
      mask TypeOptions t231_QT_dac3_datapath_mode: DUC 0 to Fs/2
      mask TypeOptions t231_QT_dac3_mixer_type: Coarse | Fine
      mask Callback t231_QT_dac3_mixer_type: mixertype_callback(gcb,231,3,'QT');
      mask TypeOptions t231_QT_dac3_mixer_mode: Real -> Real | I/Q -> Real
      mask Callback t231_QT_dac3_mixer_mode: mixer_callback(gcb,231,3,'QT')
      mask TypeOptions t231_QT_dac3_coarse_freq: 0
      mask TypeOptions t231_QT_dac3_nyquist_zone: Zone 1 | Zone 2
      mask TypeOptions t231_QT_dac3_decode_mode: SNR Optimized | Linearity Optimized
      mask Callback t231_DT_dac0_enable: enable_dac_opt(gcb,231,0,'DT');
      mask TypeOptions t231_DT_dac0_analog_output: Real | I/Q
      mask Callback t231_DT_dac0_analog_output:
      | validate_analog_data(gcb,231,0,'DT');
      | update_axis_clk(gcb,231);
      mask TypeOptions t231_DT_dac0_inter_mode: 1x | 2x | 3x | 4x | 5x | 6x | 8x | 10x | 12x | 16x | 20x | 24x | 40x
      mask Callback t231_DT_dac0_inter_mode:
      | % if I/Q output mode, need to copy interp factor before updating axis clk
      | % note only the even slice for the tile makes this check
      | if chk_param(gcb, 't231_DT_dac0_analog_output', 'I/Q')
      |   inter_mode = get_param(gcb, 't231_DT_dac0_inter_mode');
      |   set_param(gcb, 't231_DT_dac1_inter_mode', inter_mode);
      | end
      | update_axis_clk(gcb,231);
      mask TypeOptions t231_DT_dac0_sample_per_cycle: 4 | 5 | 6 | 7 | 8 | 9 | 10 | 11 | 12 | 13 | 14 | 15 | 16
      mask Callback t231_DT_dac0_sample_per_cycle:
      | % if I/Q output mode, need to copy samples per clk before updating axis clk
      | % note only the even slice for the tile makes this check
      | if chk_param(gcb, 't231_DT_dac0_analog_output', 'I/Q')
      |   spc = get_param(gcb, 't231_DT_dac0_sample_per_cycle');
      |   set_param(gcb, 't231_DT_dac1_sample_per_cycle', spc);
      | end
      | update_axis_clk_label(gcb,231);
      mask TypeOptions t231_DT_dac0_datapath_mode: DUC 0 to Fs/2
      mask TypeOptions t231_DT_dac0_mixer_type: Coarse | Fine
      mask Callback t231_DT_dac0_mixer_type: mixertype_callback(gcb,231,0,'DT');
      mask TypeOptions t231_DT_dac0_mixer_mode: Real -> Real | I/Q -> Real
      mask Callback t231_DT_dac0_mixer_mode: mixer_callback(gcb,231,0,'DT');
      mask TypeOptions t231_DT_dac0_coarse_freq: 0
      mask TypeOptions t231_DT_dac0_nyquist_zone: Zone 1 | Zone 2
      mask TypeOptions t231_DT_dac0_decode_mode: SNR Optimized | Linearity Optimized
      mask Callback t231_DT_dac1_enable: enable_dac_opt(gcb,231,1,'DT');
      mask TypeOptions t231_DT_dac1_analog_output: Real
      mask Callback t231_DT_dac1_analog_output:
      | validate_analog_data(gcb,231,1,'DT');
      | update_axis_clk(gcb,231);
      mask TypeOptions t231_DT_dac1_inter_mode: 1x | 2x | 3x | 4x | 5x | 6x | 8x | 10x | 12x | 16x | 20x | 24x | 40x
      mask Callback t231_DT_dac1_inter_mode: update_axis_clk(gcb,231);
      mask TypeOptions t231_DT_dac1_sample_per_cycle: 4 | 5 | 6 | 7 | 8 | 9 | 10 | 11 | 12 | 13 | 14 | 15 | 16
      mask Callback t231_DT_dac1_sample_per_cycle: update_axis_clk_label(gcb,231);
      mask TypeOptions t231_DT_dac1_datapath_mode: DUC 0 to Fs/2
      mask TypeOptions t231_DT_dac1_mixer_type: Coarse | Fine
      mask Callback t231_DT_dac1_mixer_type: mixertype_callback(gcb,231,1,'DT');
      mask TypeOptions t231_DT_dac1_mixer_mode: Real -> Real | I/Q -> Real
      mask Callback t231_DT_dac1_mixer_mode: mixer_callback(gcb,231,1,'DT');
      mask TypeOptions t231_DT_dac1_coarse_freq: 0
      mask TypeOptions t231_DT_dac1_nyquist_zone: Zone 1 | Zone 2
      mask TypeOptions t231_DT_dac1_decode_mode: SNR Optimized | Linearity Optimized
      mask TypeOptions t224_adc_clk_src: 224 | 225 | 226 | 227 | 228 | 229 | 230 | 231
      mask TypeOptions t224_clk_dist: None | Input Refclk | PLL Output
      mask TypeOptions t225_adc_clk_src: 224 | 225 | 226 | 227 | 228 | 229 | 230 | 231
      mask TypeOptions t225_clk_dist: None | Input Refclk | PLL Output
      mask TypeOptions t226_adc_clk_src: 224 | 225 | 226 | 227 | 228 | 229 | 230 | 231
      mask TypeOptions t226_clk_dist: None | Input Refclk | PLL Output
      mask TypeOptions t227_adc_clk_src: 224 | 225 | 226 | 227 | 228 | 229 | 230 | 231
      mask TypeOptions t227_clk_dist: None | Input Refclk | PLL Output
      mask TypeOptions t228_dac_clk_src: 224 | 225 | 226 | 227 | 228 | 229 | 230 | 231
      mask TypeOptions t228_clk_dist: None | Input Refclk | PLL Output
      mask TypeOptions t229_dac_clk_src: 224 | 225 | 226 | 227 | 228 | 229 | 230 | 231
      mask TypeOptions t229_clk_dist: None | Input Refclk | PLL Output
      mask TypeOptions t230_dac_clk_src: 224 | 225 | 226 | 227 | 228 | 229 | 230 | 231
      mask TypeOptions t230_clk_dist: None | Input Refclk | PLL Output
      mask TypeOptions t231_dac_clk_src: 224 | 225 | 226 | 227 | 228 | 229 | 230 | 231
      mask TypeOptions t231_clk_dist: None | Input Refclk | PLL Output
      mask Callback maskdoneopening:
      | %assignin('base','mask_opening',0)
      | %assignin('base','run_init',1)
      | set_param(gcb,'maskopening','0')
      | set_param(gcb,'runinit','1')
      mask DialogControl ADCTileSelect Prompt: ADC Tiles
      mask DialogControl Tile224_container Prompt: Tile 224
      mask DialogControl pll_clocking_config_224 Prompt: Clocking and PLL Configuration
      mask DialogControl t224_QuadTileConfig Prompt: Quad Tile Configuration
      mask DialogControl t224_ADCPair01 Prompt: ADC Pair 0,1
      mask DialogControl t224_QT_adc0 Prompt: ADC 0
      mask DialogControl t224_QT_adc0_DataSettings Prompt: Data Settings
      mask DialogControl t224_QT_adc0_req_axis_clk_label Prompt: Required AXI4-Stream clock:
      mask DialogControl t224_QT_adc0_MixerSettings Prompt: MIxer Settings
      mask DialogControl t224_QT_adc0_AnalogSettings Prompt: Analog Settings
      mask DialogControl t224_QT_adc1 Prompt: ADC 1
      mask DialogControl t224_QT_adc1_DataSettings Prompt: Data Settings
      mask DialogControl t224_QT_adc1_req_axis_clk_label Prompt: Required AXI4-Stream clock:
      mask DialogControl t224_QT_adc1_MixerSettings Prompt: MIxer Settings
      mask DialogControl t224_QT_adc1_AnalogSettings Prompt: Analog Settings
      mask DialogControl ADCPair23 Prompt: ADC Pair 2,3
      mask DialogControl QT_adc2 Prompt: ADC 2
      mask DialogControl t224_QT_adc2_DataSettings Prompt: Data Settings
      mask DialogControl t224_QT_adc2_req_axis_clk_label Prompt: Required AXI4-Stream clock:
      mask DialogControl t224_QT_adc2_MixerSettings Prompt: MIxer Settings
      mask DialogControl t224_QT_adc2_AnalogSettings Prompt: Analog Settings
      mask DialogControl t224_QT_adc3 Prompt: ADC 3
      mask DialogControl t224_QT_adc3_DataSettings Prompt: Data Settings
      mask DialogControl t224_QT_adc3_req_axis_clk_label Prompt: Required AXI4-Stream clock:
      mask DialogControl t224_QT_adc3_MixerSettings Prompt: MIxer Settings
      mask DialogControl t224_QT_adc3_AnalogSettings Prompt: Analog Settings
      mask DialogControl t224_DualTileConfig Prompt: Dual Tile Configuration
      mask DialogControl t224_DT_adc0 Prompt: ADC 0
      mask DialogControl t224_DT_adc0_DataSettings Prompt: Data Settings
      mask DialogControl t224_DT_adc0_req_axis_clk_label Prompt: Required AXI4-Stream clock:
      mask DialogControl t224_DT_adc0_MixerSettings Prompt: MIxer Settings
      mask DialogControl t224_DT_adc0_AnalogSettings Prompt: Analog Settings
      mask DialogControl t224_DT_adc1 Prompt: ADC 1
      mask DialogControl t224_DT_adc1_DataSettings Prompt: Data Settings
      mask DialogControl t224_DT_adc1_req_axis_clk_label Prompt: Required AXI4-Stream clock:
      mask DialogControl t224_DT_adc1_MixerSettings Prompt: MIxer Settings
      mask DialogControl t224_DT_adc1_AnalogSettings Prompt: Analog Settings
      mask DialogControl Tile225_container Prompt: Tile 225
      mask DialogControl pll_clocking_config_225 Prompt: Clocking and PLL Configuration
      mask DialogControl t225_QuadTileConfig Prompt: Quad Tile Configuration
      mask DialogControl t225_ADCPair01 Prompt: ADC Pair 0,1
      mask DialogControl t225_QT_adc0 Prompt: ADC 0
      mask DialogControl t225_QT_adc0_DataSettings Prompt: Data Settings
      mask DialogControl t225_QT_adc0_req_axis_clk_label Prompt: Required AXI4-Stream clock:
      mask DialogControl t225_QT_adc0_MixerSettings Prompt: MIxer Settings
      mask DialogControl t225_QT_adc0_AnalogSettings Prompt: Analog Settings
      mask DialogControl t225_QT_adc1 Prompt: ADC 1
      mask DialogControl t225_QT_adc1_DataSettings Prompt: Data Settings
      mask DialogControl t225_QT_adc1_req_axis_clk_label Prompt: Required AXI4-Stream clock:
      mask DialogControl t225_QT_adc1_MixerSettings Prompt: MIxer Settings
      mask DialogControl t225_QT_adc1_AnalogSettings Prompt: Analog Settings
      mask DialogControl t225_ADCPair23 Prompt: ADC Pair 2,3
      mask DialogControl t225_QT_adc2 Prompt: ADC 2
      mask DialogControl t225_QT_adc2_DataSettings Prompt: Data Settings
      mask DialogControl t225_QT_adc2_req_axis_clk_label Prompt: Required AXI4-Stream clock:
      mask DialogControl t225_QT_adc2_MixerSettings Prompt: MIxer Settings
      mask DialogControl t225_QT_adc2_AnalogSettings Prompt: Analog Settings
      mask DialogControl t225_QT_adc3 Prompt: ADC 3
      mask DialogControl t225_QT_adc3_DataSettings Prompt: Data Settings
      mask DialogControl t225_QT_adc3_req_axis_clk_label Prompt: Required AXI4-Stream clock:
      mask DialogControl t225_QT_adc3_MixerSettings Prompt: MIxer Settings
      mask DialogControl t225_QT_adc3_AnalogSettings Prompt: Analog Settings
      mask DialogControl t225_DualTileConfig Prompt: Dual Tile Configuration
      mask DialogControl t225_DT_adc0 Prompt: ADC 0
      mask DialogControl t225_DT_adc0_DataSettings Prompt: Data Settings
      mask DialogControl t225_DT_adc0_req_axis_clk_label Prompt: Required AXI4-Stream clock:
      mask DialogControl t225_DT_adc0_MixerSettings Prompt: MIxer Settings
      mask DialogControl t225_DT_adc0_AnalogSettings Prompt: Analog Settings
      mask DialogControl t225_DT_adc1 Prompt: ADC 1
      mask DialogControl t225_DT_adc1_DataSettings Prompt: Data Settings
      mask DialogControl t225_DT_adc1_req_axis_clk_label Prompt: Required AXI4-Stream clock:
      mask DialogControl t225_DT_adc1_MixerSettings Prompt: MIxer Settings
      mask DialogControl t225_DT_adc1_AnalogSettings Prompt: Analog Settings
      mask DialogControl Tile226_container Prompt: Tile 226
      mask DialogControl pll_clocking_config_226 Prompt: Clocking and PLL Configuration
      mask DialogControl t226_QuadTileConfig Prompt: Quad Tile Configuration
      mask DialogControl t226_ADCPair01 Prompt: ADC Pair 0,1
      mask DialogControl t226_QT_adc0 Prompt: ADC 0
      mask DialogControl t226_QT_adc0_DataSettings Prompt: Data Settings
      mask DialogControl t226_QT_adc0_req_axis_clk_label Prompt: Required AXI4-Stream clock:
      mask DialogControl t226_QT_adc0_MixerSettings Prompt: MIxer Settings
      mask DialogControl t226_QT_adc0_AnalogSettings Prompt: Analog Settings
      mask DialogControl t226_QT_adc1 Prompt: ADC 1
      mask DialogControl t226_QT_adc1_DataSettings Prompt: Data Settings
      mask DialogControl t226_QT_adc1_req_axis_clk_label Prompt: Required AXI4-Stream clock:
      mask DialogControl t226_QT_adc1_MixerSettings Prompt: MIxer Settings
      mask DialogControl t226_QT_adc1_AnalogSettings Prompt: Analog Settings
      mask DialogControl t226_ADCPair23 Prompt: ADC Pair 2,3
      mask DialogControl t226_QT_adc2 Prompt: ADC 2
      mask DialogControl t226_QT_adc2_DataSettings Prompt: Data Settings
      mask DialogControl t226_QT_adc2_req_axis_clk_label Prompt: Required AXI4-Stream clock:
      mask DialogControl t226_QT_adc2_MixerSettings Prompt: MIxer Settings
      mask DialogControl t226_QT_adc2_AnalogSettings Prompt: Analog Settings
      mask DialogControl t226_QT_adc3 Prompt: ADC 3
      mask DialogControl t226_QT_adc3_DataSettings Prompt: Data Settings
      mask DialogControl t226_QT_adc3_req_axis_clk_label Prompt: Required AXI4-Stream clock:
      mask DialogControl t226_QT_adc3_MixerSettings Prompt: MIxer Settings
      mask DialogControl t226_QT_adc3_AnalogSettings Prompt: Analog Settings
      mask DialogControl t226_DualTileConfig Prompt: Dual Tile Configuration
      mask DialogControl t226_DT_adc0 Prompt: ADC 0
      mask DialogControl t226_DT_adc0_DataSettings Prompt: Data Settings
      mask DialogControl t226_DT_adc0_req_axis_clk_label Prompt: Required AXI4-Stream clock:
      mask DialogControl t226_DT_adc0_MixerSettings Prompt: MIxer Settings
      mask DialogControl t226_DT_adc0_AnalogSettings Prompt: Analog Settings
      mask DialogControl t226_DT_adc1 Prompt: ADC 1
      mask DialogControl t226_DT_adc1_DataSettings Prompt: Data Settings
      mask DialogControl t226_DT_adc1_req_axis_clk_label Prompt: Required AXI4-Stream clock:
      mask DialogControl t226_DT_adc1_MixerSettings Prompt: MIxer Settings
      mask DialogControl t226_DT_adc1_AnalogSettings Prompt: Analog Settings
      mask DialogControl Tile227_container Prompt: Tile 227
      mask DialogControl pll_clocking_config_227 Prompt: Clocking and PLL Configuration
      mask DialogControl t227_QuadTileConfig Prompt: Quad Tile Configuration
      mask DialogControl t227_ADCPair01 Prompt: ADC Pair 0,1
      mask DialogControl t227_QT_adc0 Prompt: ADC 0
      mask DialogControl t227_QT_adc0_DataSettings Prompt: Data Settings
      mask DialogControl t227_QT_adc0_req_axis_clk_label Prompt: Required AXI4-Stream clock:
      mask DialogControl t227_QT_adc0_MixerSettings Prompt: MIxer Settings
      mask DialogControl t227_QT_adc0_AnalogSettings Prompt: Analog Settings
      mask DialogControl t227_QT_adc1 Prompt: ADC 1
      mask DialogControl t227_QT_adc1_DataSettings Prompt: Data Settings
      mask DialogControl t227_QT_adc1_req_axis_clk_label Prompt: Required AXI4-Stream clock:
      mask DialogControl t227_QT_adc1_MixerSettings Prompt: MIxer Settings
      mask DialogControl t227_QT_adc1_AnalogSettings Prompt: Analog Settings
      mask DialogControl t227_ADCPair23 Prompt: ADC Pair 2,3
      mask DialogControl t227_QT_adc2 Prompt: ADC 2
      mask DialogControl t227_QT_adc2_DataSettings Prompt: Data Settings
      mask DialogControl t227_QT_adc2_req_axis_clk_label Prompt: Required AXI4-Stream clock:
      mask DialogControl t227_QT_adc2_MixerSettings Prompt: MIxer Settings
      mask DialogControl t227_QT_adc2_AnalogSettings Prompt: Analog Settings
      mask DialogControl t227_QT_adc3 Prompt: ADC 3
      mask DialogControl t227_QT_adc3_DataSettings Prompt: Data Settings
      mask DialogControl t227_QT_adc3_req_axis_clk_label Prompt: Required AXI4-Stream clock:
      mask DialogControl t227_QT_adc3_MixerSettings Prompt: MIxer Settings
      mask DialogControl t227_QT_adc3_AnalogSettings Prompt: Analog Settings
      mask DialogControl t227_DualTileConfig Prompt: Dual Tile Configuration
      mask DialogControl t227_DT_adc0 Prompt: ADC 0
      mask DialogControl t227_DT_adc0_DataSettings Prompt: Data Settings
      mask DialogControl t227_DT_adc0_req_axis_clk_label Prompt: Required AXI4-Stream clock:
      mask DialogControl t227_DT_adc0_MixerSettings Prompt: MIxer Settings
      mask DialogControl t227_DT_adc0_AnalogSettings Prompt: Analog Settings
      mask DialogControl t227_DT_adc1 Prompt: ADC 1
      mask DialogControl t227_DT_adc1_DataSettings Prompt: Data Settings
      mask DialogControl t227_DT_adc1_req_axis_clk_label Prompt: Required AXI4-Stream clock:
      mask DialogControl t227_DT_adc1_MixerSettings Prompt: MIxer Settings
      mask DialogControl t227_DT_adc1_AnalogSettings Prompt: Analog Settings
      mask DialogControl DACTileSelect Prompt: DAC Tiles
      mask DialogControl Tile228_container Prompt: Tile 228
      mask DialogControl pll_clocking_config_228 Prompt: Clocking and PLL Configuration
      mask DialogControl t228_QuadTileConfig Prompt: Quad Tile Configuration
      mask DialogControl t228_DACPair01 Prompt: DAC Pair 0,1
      mask DialogControl t228_QT_dac0 Prompt: DAC 0
      mask DialogControl t228_QT_dac0_DataSettings Prompt: Data Settings
      mask DialogControl t228_QT_dac0_req_axis_clk_label Prompt: Required AXI4-Stream clock:
      mask DialogControl t228_QT_dac0_MixerSettings Prompt: MIxer Settings
      mask DialogControl t228_QT_dac0_AnalogSettings Prompt: Analog Settings
      mask DialogControl t228_QT_dac1 Prompt: DAC 1
      mask DialogControl t228_QT_dac1_DataSettings Prompt: Data Settings
      mask DialogControl t228_QT_dac1_req_axis_clk_label Prompt: Required AXI4-Stream clock:
      mask DialogControl t228_QT_dac1_MixerSettings Prompt: MIxer Settings
      mask DialogControl t228_QT_dac1_AnalogSettings Prompt: Analog Settings
      mask DialogControl t228_DACPair23 Prompt: DAC Pair 2,3
      mask DialogControl t228_QT_dac2 Prompt: DAC 2
      mask DialogControl t228_QT_dac2_DataSettings Prompt: Data Settings
      mask DialogControl t228_QT_dac2_req_axis_clk_label Prompt: Required AXI4-Stream clock:
      mask DialogControl t228_QT_dac2_MixerSettings Prompt: MIxer Settings
      mask DialogControl t228_QT_dac2_AnalogSettings Prompt: Analog Settings
      mask DialogControl t228_QT_dac3 Prompt: DAC 3
      mask DialogControl t228_QT_dac3_DataSettings Prompt: Data Settings
      mask DialogControl t228_QT_dac3_req_axis_clk_label Prompt: Required AXI4-Stream clock:
      mask DialogControl t228_QT_dac3_MixerSettings Prompt: MIxer Settings
      mask DialogControl t228_QT_dac3_AnalogSettings Prompt: Analog Settings
      mask DialogControl t228_DualTileConfig Prompt: Dual Tile Configuration
      mask DialogControl t228_DT_dac0 Prompt: DAC 0
      mask DialogControl t228_DT_dac0_DataSettings Prompt: Data Settings
      mask DialogControl t228_DT_dac0_req_axis_clk_label Prompt: Required AXI4-Stream clock:
      mask DialogControl t228_DT_dac0_MixerSettings Prompt: MIxer Settings
      mask DialogControl t228_DT_dac0_AnalogSettings Prompt: Analog Settings
      mask DialogControl t228_DT_dac1 Prompt: DAC 1
      mask DialogControl t228_DT_dac1_DataSettings Prompt: Data Settings
      mask DialogControl t228_DT_dac1_req_axis_clk_label Prompt: Required AXI4-Stream clock:
      mask DialogControl t228_DT_dac1_MixerSettings Prompt: MIxer Settings
      mask DialogControl t228_DT_dac1_AnalogSettings Prompt: Analog Settings
      mask DialogControl Tile229_container Prompt: Tile 229
      mask DialogControl pll_clocking_config_229 Prompt: Clocking and PLL Configuration
      mask DialogControl t229_QuadTileConfig Prompt: Quad Tile Configuration
      mask DialogControl t229_DACPair01 Prompt: DAC Pair 0,1
      mask DialogControl t229_QT_dac0 Prompt: DAC 0
      mask DialogControl t229_QT_dac0_DataSettings Prompt: Data Settings
      mask DialogControl t229_QT_dac0_req_axis_clk_label Prompt: Required AXI4-Stream clock:
      mask DialogControl t229_QT_dac0_MixerSettings Prompt: MIxer Settings
      mask DialogControl t229_QT_dac0_AnalogSettings Prompt: Analog Settings
      mask DialogControl t229_QT_dac1 Prompt: DAC 1
      mask DialogControl t229_QT_dac1_DataSettings Prompt: Data Settings
      mask DialogControl t229_QT_dac1_req_axis_clk_label Prompt: Required AXI4-Stream clock:
      mask DialogControl t229_QT_dac1_MixerSettings Prompt: MIxer Settings
      mask DialogControl t229_QT_dac1_AnalogSettings Prompt: Analog Settings
      mask DialogControl t229_DACPair23 Prompt: DAC Pair 2,3
      mask DialogControl t229_QT_dac2 Prompt: DAC 2
      mask DialogControl t229_QT_dac2_DataSettings Prompt: Data Settings
      mask DialogControl t229_QT_dac2_req_axis_clk_label Prompt: Required AXI4-Stream clock:
      mask DialogControl t229_QT_dac2_MixerSettings Prompt: MIxer Settings
      mask DialogControl t229_QT_dac2_AnalogSettings Prompt: Analog Settings
      mask DialogControl t229_QT_dac3 Prompt: DAC 3
      mask DialogControl t229_QT_dac3_DataSettings Prompt: Data Settings
      mask DialogControl t229_QT_dac3_req_axis_clk_label Prompt: Required AXI4-Stream clock:
      mask DialogControl t229_QT_dac3_MixerSettings Prompt: MIxer Settings
      mask DialogControl t229_QT_dac3_AnalogSettings Prompt: Analog Settings
      mask DialogControl t229_DualTileConfig Prompt: Dual Tile Configuration
      mask DialogControl t229_DT_dac0 Prompt: DAC 0
      mask DialogControl t229_DT_dac0_DataSettings Prompt: Data Settings
      mask DialogControl t229_DT_dac0_req_axis_clk_label Prompt: Required AXI4-Stream clock:
      mask DialogControl t229_DT_dac0_MixerSettings Prompt: MIxer Settings
      mask DialogControl t229_DT_dac0_AnalogSettings Prompt: Analog Settings
      mask DialogControl t229_DT_dac1 Prompt: DAC 1
      mask DialogControl t229_DT_dac1_DataSettings Prompt: Data Settings
      mask DialogControl t229_DT_dac1_req_axis_clk_label Prompt: Required AXI4-Stream clock:
      mask DialogControl t229_DT_dac1_MixerSettings Prompt: MIxer Settings
      mask DialogControl t229_DT_dac1_AnalogSettings Prompt: Analog Settings
      mask DialogControl Tile230_container Prompt: Tile 230
      mask DialogControl pll_clocking_config_230 Prompt: Clocking and PLL Configuration
      mask DialogControl t230_QuadTileConfig Prompt: Quad Tile Configuration
      mask DialogControl t230_DACPair01 Prompt: DAC Pair 0,1
      mask DialogControl t230_QT_dac0 Prompt: DAC 0
      mask DialogControl t230_QT_dac0_DataSettings Prompt: Data Settings
      mask DialogControl t230_QT_dac0_req_axis_clk_label Prompt: Required AXI4-Stream clock:
      mask DialogControl t230_QT_dac0_MixerSettings Prompt: MIxer Settings
      mask DialogControl t230_QT_dac0_AnalogSettings Prompt: Analog Settings
      mask DialogControl t230_QT_dac1 Prompt: DAC 1
      mask DialogControl t230_QT_dac1_DataSettings Prompt: Data Settings
      mask DialogControl t230_QT_dac1_req_axis_clk_label Prompt: Required AXI4-Stream clock:
      mask DialogControl t230_QT_dac1_MixerSettings Prompt: MIxer Settings
      mask DialogControl t230_QT_dac1_AnalogSettings Prompt: Analog Settings
      mask DialogControl t230_DACPair23 Prompt: DAC Pair 2,3
      mask DialogControl t230_QT_dac2 Prompt: DAC 2
      mask DialogControl t230_QT_dac2_DataSettings Prompt: Data Settings
      mask DialogControl t230_QT_dac2_req_axis_clk_label Prompt: Required AXI4-Stream clock:
      mask DialogControl t230_QT_dac2_MixerSettings Prompt: MIxer Settings
      mask DialogControl t230_QT_dac2_AnalogSettings Prompt: Analog Settings
      mask DialogControl t230_QT_dac3 Prompt: DAC 3
      mask DialogControl t230_QT_dac3_DataSettings Prompt: Data Settings
      mask DialogControl t230_QT_dac3_req_axis_clk_label Prompt: Required AXI4-Stream clock:
      mask DialogControl t230_QT_dac3_MixerSettings Prompt: MIxer Settings
      mask DialogControl t230_QT_dac3_AnalogSettings Prompt: Analog Settings
      mask DialogControl t230_DualTileConfig Prompt: Dual Tile Configuration
      mask DialogControl t230_DT_dac0 Prompt: DAC 0
      mask DialogControl t230_DT_dac0_DataSettings Prompt: Data Settings
      mask DialogControl t230_DT_dac0_req_axis_clk_label Prompt: Required AXI4-Stream clock:
      mask DialogControl t230_DT_dac0_MixerSettings Prompt: MIxer Settings
      mask DialogControl t230_DT_dac0_AnalogSettings Prompt: Analog Settings
      mask DialogControl t230_DT_dac1 Prompt: DAC 1
      mask DialogControl t230_DT_dac1_DataSettings Prompt: Data Settings
      mask DialogControl t230_DT_dac1_req_axis_clk_label Prompt: Required AXI4-Stream clock:
      mask DialogControl t230_DT_dac1_MixerSettings Prompt: MIxer Settings
      mask DialogControl t230_DT_dac1_AnalogSettings Prompt: Analog Settings
      mask DialogControl Tile231_container Prompt: Tile 231
      mask DialogControl pll_clocking_config_231 Prompt: Clocking and PLL Configuration
      mask DialogControl t231_QuadTileConfig Prompt: Quad Tile Configuration
      mask DialogControl t231_DACPair01 Prompt: DAC Pair 0,1
      mask DialogControl t231_QT_dac0 Prompt: DAC 0
      mask DialogControl t231_QT_dac0_DataSettings Prompt: Data Settings
      mask DialogControl t231_QT_dac0_req_axis_clk_label Prompt: Required AXI4-Stream clock:
      mask DialogControl t231_QT_dac0_MixerSettings Prompt: MIxer Settings
      mask DialogControl t231_QT_dac0_AnalogSettings Prompt: Analog Settings
      mask DialogControl t231_QT_dac1 Prompt: DAC 1
      mask DialogControl t231_QT_dac1_DataSettings Prompt: Data Settings
      mask DialogControl t231_QT_dac1_req_axis_clk_label Prompt: Required AXI4-Stream clock:
      mask DialogControl t231_QT_dac1_MixerSettings Prompt: MIxer Settings
      mask DialogControl t231_QT_dac1_AnalogSettings Prompt: Analog Settings
      mask DialogControl t231_DACPair23 Prompt: DAC Pair 2,3
      mask DialogControl t231_QT_dac2 Prompt: DAC 2
      mask DialogControl t231_QT_dac2_DataSettings Prompt: Data Settings
      mask DialogControl t231_QT_dac2_req_axis_clk_label Prompt: Required AXI4-Stream clock:
      mask DialogControl t231_QT_dac2_MixerSettings Prompt: MIxer Settings
      mask DialogControl t231_QT_dac2_AnalogSettings Prompt: Analog Settings
      mask DialogControl t231_QT_dac3 Prompt: DAC 3
      mask DialogControl t231_QT_dac3_DataSettings Prompt: Data Settings
      mask DialogControl t231_QT_dac3_req_axis_clk_label Prompt: Required AXI4-Stream clock:
      mask DialogControl t231_QT_dac3_MixerSettings Prompt: MIxer Settings
      mask DialogControl t231_QT_dac3_AnalogSettings Prompt: Analog Settings
      mask DialogControl t231_DualTileConfig Prompt: Dual Tile Configuration
      mask DialogControl t231_DT_dac0 Prompt: DAC 0
      mask DialogControl t231_DT_dac0_DataSettings Prompt: Data Settings
      mask DialogControl t231_DT_dac0_req_axis_clk_label Prompt: Required AXI4-Stream clock:
      mask DialogControl t231_DT_dac0_MixerSettings Prompt: MIxer Settings
      mask DialogControl t231_DT_dac0_AnalogSettings Prompt: Analog Settings
      mask DialogControl t231_DT_dac1 Prompt: DAC 1
      mask DialogControl t231_DT_dac1_DataSettings Prompt: Data Settings
      mask DialogControl t231_DT_dac1_req_axis_clk_label Prompt: Required AXI4-Stream clock:
      mask DialogControl t231_DT_dac1_MixerSettings Prompt: MIxer Settings
      mask DialogControl t231_DT_dac1_AnalogSettings Prompt: Analog Settings
      mask DialogControl SystemClocking Prompt: System Clocking And Real-time Ports
      mask DialogControl ADCClocking Prompt: ADC Tile Clocking
      mask DialogControl t224_clock_config Prompt: ADC Tile 224
      mask DialogControl t225_clock_config Prompt: ADC Tile 225
      mask DialogControl t226_clock_config Prompt: ADC Tile 226
      mask DialogControl t227_clock_config Prompt: ADC Tile 227
      mask DialogControl DACClocking Prompt: DAC Tile Clocking
      mask DialogControl t228_clock_config Prompt: DAC Tile 228
      mask DialogControl t229_clock_config Prompt: DAC Tile 229
      mask DialogControl t230_clock_config Prompt: DAC Tile 230
      mask DialogControl t231_clock_config Prompt: DAC Tile 231
  simple_bram_vacc : Subsystem  AncestorBlock=casper_library_accumulators/simple_bram_vacc  mask(simple_bram_vacc){vec_len=512, arith_type=Unsigned, n_bits=64, bin_pt=34}
      mask prompts: vec_len "Vector length:"; arith_type "Output type:"; n_bits "Bit width (output):"; bin_pt "Binary point (output):"
      mask help: This simple vector accumulator is based on a shift register. It outputs its previous accumulated vector after a new_acc pulse is received.
      mask init:
      | simple_bram_vacc_init(gcb, ...
      |     'vec_len', vec_len, ...
      |     'arith_type', arith_type, ...
      |     'n_bits', n_bits, ...
      |     'bin_pt', bin_pt);
      mask TypeOptions arith_type: Signed | Unsigned
  simple_bram_vacc1 : Subsystem  AncestorBlock=casper_library_accumulators/simple_bram_vacc  mask(simple_bram_vacc){vec_len=512, arith_type=Unsigned, n_bits=64, bin_pt=34}
      mask prompts: vec_len "Vector length:"; arith_type "Output type:"; n_bits "Bit width (output):"; bin_pt "Binary point (output):"
      mask help: This simple vector accumulator is based on a shift register. It outputs its previous accumulated vector after a new_acc pulse is received.
      mask init:
      | simple_bram_vacc_init(gcb, ...
      |     'vec_len', vec_len, ...
      |     'arith_type', arith_type, ...
      |     'n_bits', n_bits, ...
      |     'bin_pt', bin_pt);
      mask TypeOptions arith_type: Signed | Unsigned
  simple_bram_vacc2 : Subsystem  AncestorBlock=casper_library_accumulators/simple_bram_vacc  mask(simple_bram_vacc){vec_len=512, arith_type=Unsigned, n_bits=64, bin_pt=34}
      mask prompts: vec_len "Vector length:"; arith_type "Output type:"; n_bits "Bit width (output):"; bin_pt "Binary point (output):"
      mask help: This simple vector accumulator is based on a shift register. It outputs its previous accumulated vector after a new_acc pulse is received.
      mask init:
      | simple_bram_vacc_init(gcb, ...
      |     'vec_len', vec_len, ...
      |     'arith_type', arith_type, ...
      |     'n_bits', n_bits, ...
      |     'bin_pt', bin_pt);
      mask TypeOptions arith_type: Signed | Unsigned
  simple_bram_vacc3 : Subsystem  AncestorBlock=casper_library_accumulators/simple_bram_vacc  mask(simple_bram_vacc){vec_len=512, arith_type=Unsigned, n_bits=64, bin_pt=34}
      mask prompts: vec_len "Vector length:"; arith_type "Output type:"; n_bits "Bit width (output):"; bin_pt "Binary point (output):"
      mask help: This simple vector accumulator is based on a shift register. It outputs its previous accumulated vector after a new_acc pulse is received.
      mask init:
      | simple_bram_vacc_init(gcb, ...
      |     'vec_len', vec_len, ...
      |     'arith_type', arith_type, ...
      |     'n_bits', n_bits, ...
      |     'bin_pt', bin_pt);
      mask TypeOptions arith_type: Signed | Unsigned
  snapshot_ctrl : Subsystem  Tag=xps:sw_reg  AncestorBlock=xps_library/Memory/software_register  mask(swreg){io_dir=From Processor, io_delay=0, init_val=0, sample_period=1, names=[start], bitwidths=1, bin_pts=0, arith_types=2, sim_port=on, show_format=on}
      mask prompts: io_dir "I/O direction"; io_delay "I/O delay"; init_val "Initial Value"; sample_period "Sample period"; names "Bitfield names [msb...lsb]"; bitwidths "Bitfield widths"; bin_pts "Bitfield binary pts"; arith_types "Bitfield types, ufix=0, fix=1, bool=2"; sim_port "Provide sim input/output?"; show_format "Print format string?"
      mask help: A 32-bit software-accessible register. Can be divided into bitfields of varying widths and types using the fields in the block mask.
      mask init:
      | swreg_init(gcb)
      settings: AttributesFormatString=1input:b = 1 bits
      mask TypeOptions io_dir: To Processor | From Processor
      mask Callback io_dir:
      | mask_enables = get_param(gcb, 'MaskEnables');
      | mask_names = get_param(gcb, 'MaskNames');
      | if strcmp(get_param(gcb, 'io_dir'), 'To Processor'),
      |     mask_enables{ismember(mask_names, 'sample_period')} = 'off';
      | else
      |     mask_enables{ismember(mask_names, 'sample_period')} = 'on';
      | end
      | set_param(gcb, 'MaskEnables', mask_enables);
      mask DialogControl ParameterTabVar0 Prompt: Setup
  spect_cnt : hdlBasic/Counter  cnt_type=Free running  cnt_to=Inf  operation=Up  start_count=0  cnt_by_val=1  arith_type=Unsigned  n_bits=9  bin_pt=0  load_pin=off  rst=on  en=on  explicit_period=Explicit  period=1  use_behavioral_HDL=off  implementation=Fabric  use_rpm=off  XmcBlockStatus=1  maskContainerNames=group1  block_type=counter  block_config=sysgen:Counter_config  block_width=531  block_height=1023
  sync_cnt : Subsystem  Tag=xps:sw_reg  AncestorBlock=xps_library/Memory/software_register  mask(swreg){io_dir=To Processor, io_delay=0, init_val=0, sample_period=1, names=reg, bitwidths=32, bin_pts=0, arith_types=0, sim_port=on, show_format=off}
      mask prompts: io_dir "I/O direction"; io_delay "I/O delay"; init_val "Initial Value"; sample_period "Sample period"; names "Bitfield names [msb...lsb]"; bitwidths "Bitfield widths"; bin_pts "Bitfield binary pts"; arith_types "Bitfield types, ufix=0, fix=1, bool=2"; sim_port "Provide sim input/output?"; show_format "Print format string?"
      mask help: A 32-bit software-accessible register. Can be divided into bitfields of varying widths and types using the fields in the block mask.
      mask init:
      | swreg_init(gcb)
      settings: AttributesFormatString=1output
      mask TypeOptions io_dir: To Processor | From Processor
      mask Callback io_dir:
      | mask_enables = get_param(gcb, 'MaskEnables');
      | mask_names = get_param(gcb, 'MaskNames');
      | if strcmp(get_param(gcb, 'io_dir'), 'To Processor'),
      |     mask_enables{ismember(mask_names, 'sample_period')} = 'off';
      | else
      |     mask_enables{ismember(mask_names, 'sample_period')} = 'on';
      | end
      | set_param(gcb, 'MaskEnables', mask_enables);
      mask DialogControl ParameterTabVar0 Prompt: Setup
  sync_cntr : hdlBasic/Counter  cnt_type=Free running  cnt_to=Inf  operation=Up  start_count=0  cnt_by_val=1  arith_type=Unsigned  n_bits=32  bin_pt=0  load_pin=off  rst=on  en=on  explicit_period=Explicit  period=1  use_behavioral_HDL=off  implementation=Fabric  use_rpm=off  XmcBlockStatus=1  maskContainerNames=group1  block_type=counter  block_config=sysgen:Counter_config  block_width=531  block_height=1023
  sync_gen : Subsystem  AncestorBlock=casper_library_misc/sync_gen  mask(sync_gen){sim_acc_len=1, fft_size=2048, fft_simult_inputs=4, pfb_fir_taps=4, reorder_vec=[2 2 9], scale=2048}
      mask prompts: sim_acc_len "Simulation Accumulation Length"; fft_size "FFT Size"; fft_simult_inputs "Simultaneous Inputs (FFT)"; pfb_fir_taps "Taps in pfb_fir (use 1 if no pfb_fir)"; reorder_vec "Reorder Orders (e.g. [2 2 2])"
      mask help:
      | This block computes the sync period based on system parameters as
      | described in Casper memo.  Detailed descritions of the block's
      | variables can be found in the 'Block Documentation' section of
      | the CASPER wiki.
      mask init:
      | sync_gen_init(gcb, ...
      |     'sim_acc_len', sim_acc_len, ...
      |     'fft_size', fft_size, ...
      |     'fft_simult_inputs', fft_simult_inputs,...
      |     'pfb_fir_taps', pfb_fir_taps, ...
      |     'reorder_vec', reorder_vec, ...
      |     'scale', scale);
      settings: AttributesFormatString=sim_sync_period=75497472
      mask Help:
      | SyncPeriod=LCM(reorder_vec)*(acc_num)*(pfb_fir_len)*(fft_size/fft_simult_inputs)
      | 
      | See CASPER sync pulse memo for more details.
  wires:
  led0_sync/1 -> Terminator20/1
  pulse_ext1/1(out) -> pipeline1/1(d)
  pipeline3/1(q) -> pfb_fir/1(sync)
  sync_cntr/1 -> Delay21/1
  cnt_rst/1(in_reg) -> pipeline9/1(d)
  Constant19/1 -> cnt_rst/1(sim_1)
  sync_cnt/1(sim_out_reg) -> Terminator7/1
  led1_new_acc/1 -> Terminator24/1
  pulse_ext2/1(out) -> pipeline20/1(d)
  Constant16/1 -> acc_len/1(sim_1)
  acc_len/1(in_reg) -> pipeline8/1(d)
  acc_cntr/1 -> Delay1/1
  acc_cnt/1(sim_out_reg) -> Terminator1/1
  Delay1/1 -> acc_cnt/1(out_reg)
  [cnt_rst] -> acc_cntr/1
  pipeline9/1(q) -> Slice2/1
  Delay21/1 -> sync_cnt/1(out_reg)
  Delay28/1 -> acc_cntr/2
  pipeline20/1(q) -> led1_new_acc/1
  pipeline19/1(q) -> pulse_ext2/1(in)
  [cnt_rst] -> sync_cntr/1
  Slice2/1 -> [cnt_rst]
  sync_gen/1(sync_out) -> Delay23/1
  [sync_gen] -> pipeline3/1(d)
  [sync_gen] -> pipeline/1(d)
  [sync_gen] -> sync_cntr/2
  [new_acc] -> Delay28/1
  [new_acc] -> pipeline19/1(d)
  pipeline8/1(q) -> [acc_len]
  Gateway Out23/1 -> Scope2/1
  pipeline/1(q) -> pulse_ext1/1(in)
  pipeline1/1(q) -> led0_sync/1
  Delay23/1 -> [sync_gen], Gateway Out23/1
  adc_chan_sel/1(in_reg) -> Mux/1
  Mux/1 -> munge/1(din)
  munge/1(dout) -> Reinterpret9/1, bus_expand/1(bus_in)
  bus_expand/1(msb_out4) -> pfb_fir/2(pol1_in1)
  bus_expand/2(out3) -> pfb_fir/3(pol1_in2)
  bus_expand/3(out2) -> pfb_fir/4(pol1_in3)
  bus_expand/4(lsb_out1) -> pfb_fir/5(pol1_in4)
  pfb_fir/2(pol1_out1) -> fft/3(in00)
  pfb_fir/3(pol1_out2) -> fft/4(in01)
  pfb_fir/4(pol1_out3) -> fft/5(in02)
  pfb_fir/5(pol1_out4) -> fft/6(in03)
  pfb_fir/1(sync_out) -> fft/1(sync)
  Constant2/1 -> fft/2(shift)
  [new_acc] -> pipeline29/1(d)
  Delay6/1 -> Delay7/1
  [acc_len] -> acc_cntrl/1(acc_len)
  Delay10/1 -> Delay34/1
  power2/1 -> Delay26/1
  Delay17/1 -> power2/1
  Delay2/1 -> Delay3/1
  acc_cntrl/1(new_acc) -> [new_acc]
  Delay14/1 -> Delay10/1
  Delay26/1 -> pipeline10/1(d)
  pipeline4/1(q) -> pipeline6/1(d)
  Delay3/1 -> power3/1
  pipeline13/1(q) -> simple_bram_vacc/2(din)
  [new_acc] -> pipeline14/1(d)
  Delay16/1 -> Delay17/1
  Delay4/1 -> pipeline4/1(d)
  Delay34/1 -> Delay24/1
  Delay5/1 -> power1/1
  pipeline2/1(q) -> pipeline13/1(d)
  pipeline10/1(q) -> pipeline15/1(d)
  power4/1 -> Delay8/1
  power3/1 -> Delay4/1
  Delay24/1 -> acc_cntrl/2(sync)
  Delay25/1 -> pipeline2/1(d)
  Delay15/1 -> Delay5/1
  Delay8/1 -> pipeline28/1(d)
  pipeline28/1(q) -> pipeline30/1(d)
  [cnt_rst] -> acc_cntrl/3(rst)
  power1/1 -> Delay25/1
  [new_acc] -> pipeline5/1(d)
  Delay7/1 -> power4/1
  [new_acc] -> pipeline12/1(d)
  pipeline12/1(q) -> simple_bram_vacc/1(new_acc)
  fft/5(out03) -> Delay6/1
  fft/4(out02) -> Delay2/1
  fft/3(out01) -> Delay16/1
  fft/2(out00) -> Delay15/1
  fft/1(sync_out) -> Delay14/1
  Constant4/1 -> snapshot_ctrl/1(sim_1)
  adc_snapshot/1(arm_out) -> Terminator4/1
  snapshot_ctrl/1(in_start) -> edge_detect1/1
  edge_detect1/1 -> adc_snapshot/3(trig)
  Constant/1 -> adc_snapshot/2(we)
  fft/6(of) -> Terminator5/1
  Constant1/1 -> adc_chan_sel/1(sim_1)
  Reinterpret9/1 -> adc_snapshot/1(in_d)
  pipeline18/1(q) -> q3/3(we)
  q1/1(data_out) -> Terminator13/1
  q3/1(data_out) -> Terminator2/1
  simple_bram_vacc3/1(dout) -> Reinterpret2/1
  Reinterpret1/1 -> pipeline7/1(d)
  simple_bram_vacc/2(valid) -> pipeline25/1(d), spect_cnt/2
  pipeline27/1(q) -> q4/1(addr)
  pipeline22/1(q) -> q4/3(we)
  simple_bram_vacc2/1(dout) -> Reinterpret1/1
  pipeline23/1(q) -> q2/1(addr)
  pipeline16/1(q) -> q2/2(data_in)
  Reinterpret5/1 -> pipeline16/1(d)
  q2/1(data_out) -> Terminator14/1
  Reinterpret4/1 -> pipeline24/1(d)
  Reinterpret2/1 -> pipeline31/1(d)
  q4/1(data_out) -> Terminator3/1
  pipeline21/1(q) -> q3/1(addr)
  simple_bram_vacc1/2(valid) -> pipeline17/1(d)
  pipeline26/1(q) -> q1/1(addr)
  pipeline24/1(q) -> q1/2(data_in)
  simple_bram_vacc1/1(dout) -> Reinterpret5/1
  simple_bram_vacc3/2(valid) -> pipeline22/1(d)
  simple_bram_vacc/1(dout) -> Reinterpret4/1
  simple_bram_vacc2/2(valid) -> pipeline18/1(d)
  spect_cnt/1 -> pipeline27/1(d), pipeline21/1(d), pipeline23/1(d), pipeline26/1(d)
  pipeline31/1(q) -> q4/2(data_in)
  pipeline17/1(q) -> q2/3(we)
  pipeline7/1(q) -> q3/2(data_in)
  pipeline25/1(q) -> q1/3(we)
  pipeline14/1(q) -> simple_bram_vacc1/1(new_acc)
  pipeline15/1(q) -> simple_bram_vacc1/2(din)
  pipeline5/1(q) -> simple_bram_vacc2/1(new_acc)
  pipeline6/1(q) -> simple_bram_vacc2/2(din)
  pipeline29/1(q) -> simple_bram_vacc3/1(new_acc)
  pipeline30/1(q) -> simple_bram_vacc3/2(din)
  [new_acc] -> pipeline11/1(d)
  pipeline11/1(q) -> spect_cnt/1
  Band-Limited White Noise/1 -> rfdc/4(m30_axis_tdata_sim), rfdc/3(m20_axis_tdata_sim), rfdc/2(m10_axis_tdata_sim), rfdc/1(m00_axis_tdata_sim)
  rfdc/1(m00_axis_tdata) -> Mux/2
  rfdc/2(m10_axis_tdata) -> Mux/3
  rfdc/3(m20_axis_tdata) -> Mux/4
  rfdc/4(m30_axis_tdata) -> Mux/5
